simulink model "untitled134"  (R2019a)
settings: Solver=VariableStepAuto  StartTime=0.0  StopTime=10.0  RelTol=1e-3
settings Model: Creator=wilso  LastModifiedBy=wilso

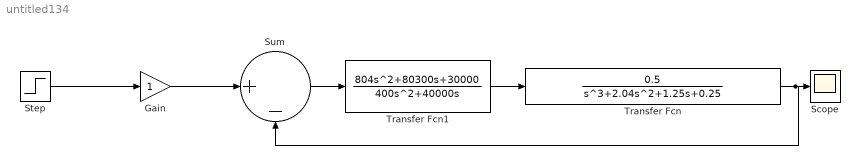
== system untitled134 ==
  Gain : Gain
  Scope : Scope
  Step : Step  SampleTime=0
  Sum : Sum  Inputs=|+-
  Transfer Fcn : TransferFcn  Numerator=[0.5]  Denominator=[1 2.04 1.25 0.25]
  Transfer Fcn1 : TransferFcn  Numerator=[804 80300 30000]  Denominator=[400 40000 0]
  wires:
  Step/1 -> Gain/1
  Gain/1 -> Sum/1
  Sum/1 -> Transfer Fcn1/1
  Transfer Fcn1/1 -> Transfer Fcn/1
  Transfer Fcn/1 -> Scope/1, Sum/2
